simulink model "step1"  (R2015b)
settings: Solver=FixedStepAuto  StartTime=0.0  StopTime=1e-5  FixedStep=1e-8  RelTol=1e-3
libraries: commsynccomp2 x1, dsparch4 x1, rfmathmodels1 x1, rfprivate1 x1
settings Model: Creator=dimple  LastModifiedBy=dimple

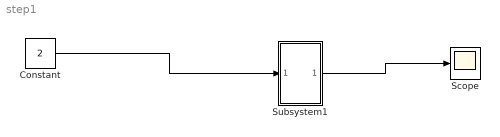
== system step1 ==
  Constant : Constant  Value=2  SampleTime=-1
  Scope : Scope
  Subsystem1 : Subsystem
  wires:
  Constant/1 -> Subsystem1/1("In1 ")
  Subsystem1/1(Out1) -> Scope/1

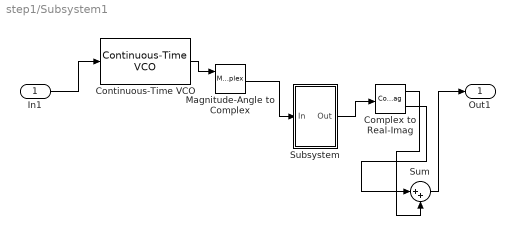
== system step1/Subsystem1 ==
  "In1 " : Inport
  Complex to Real-Imag : ComplexToRealImag
  Continuous-Time VCO : commsynccomp2/Continuous-Time VCO  Ac=10  Fc=1e6  Kc=1e5  Ph=0
  Magnitude-Angle to Complex : MagnitudeAngleToComplex
  Subsystem : Subsystem
  Sum : Sum  Inputs=|++
  Out1 : Outport
  wires:
  "In1 "/1 -> Continuous-Time VCO/1
  Subsystem/1(Out) -> Complex to Real-Imag/1
  Continuous-Time VCO/1 -> Magnitude-Angle to Complex/1
  Complex to Real-Imag/2 -> Sum/1
  Magnitude-Angle to Complex/1 -> Subsystem/1(In)
  Sum/1 -> Out1/1
  Complex to Real-Imag/1 -> Sum/2

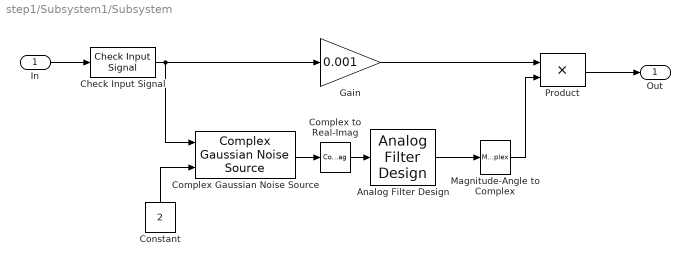
== system step1/Subsystem1/Subsystem ==
  In : Inport
  Analog Filter Design : dsparch4/Analog Filter Design  method=Butterworth  filttype=Lowpass  N=5  Wlo=1e7  Whi=80  Rp=2  Rs=40
  Check Input Signal : rfmathmodels1/Mixer/Check Input Signal  SystemSampleTime=-1
  Complex Gaussian Noise Source : rfprivate1/Complex Gaussian Noise Source  myseed=2137
  Complex to Real-Imag : ComplexToRealImag  Output=Real
  Constant : Constant  Value=2  SampleTime=Inf
  Gain : Gain  Gain=0.001  SaturateOnIntegerOverflow=on  OutDataTypeStr=Inherit: Same as input  ParamDataTypeStr=Inherit: Same as input
  Magnitude-Angle to Complex : MagnitudeAngleToComplex  Input=Angle  ConstantPart=1
  Product : Product  SaturateOnIntegerOverflow=on  InputSameDT=on  OutDataTypeStr=Inherit: Same as first input
  Out : Outport
  wires:
  Constant/1 -> Complex Gaussian Noise Source/2
  Complex Gaussian Noise Source/1 -> Complex to Real-Imag/1
  Gain/1 -> Product/1
  Check Input Signal/1 -> Complex Gaussian Noise Source/1, Gain/1
  In/1 -> Check Input Signal/1
  Product/1 -> Out/1
  Complex to Real-Imag/1 -> Analog Filter Design/1
  Magnitude-Angle to Complex/1 -> Product/2
  Analog Filter Design/1 -> Magnitude-Angle to Complex/1
